simulink model "model5"  (R2022a)
settings: Solver=FixedStepAuto  StartTime=0.0  StopTime=300  FixedStep=1  RelTol=1e-3
values from neighbouring files (symbols this model uses):
  testMap = [0  0  0; 0  1  0; 0  0  0]    [aufgabe2.mat]
settings Model: Creator=JadKHaddad  LastModifiedBy=JadKHaddad

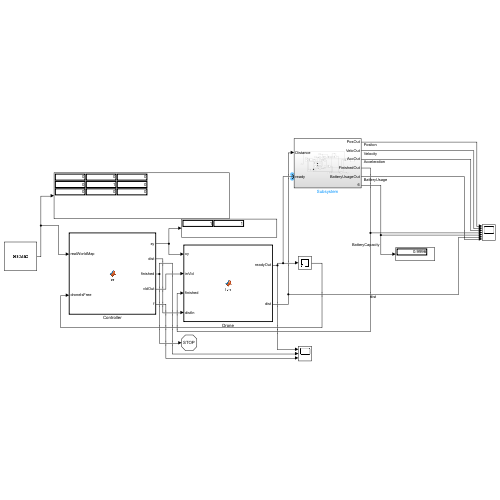
[thumbnail: Simulink's stored preview of the top-level diagram]
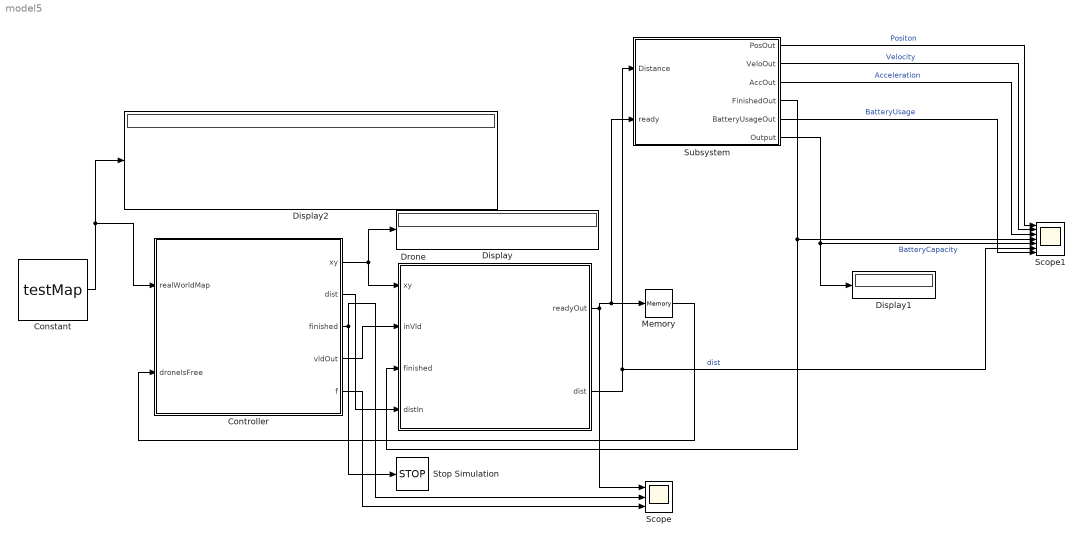
== system model5 ==
  Constant : Constant  Value=testMap  VectorParams1D=off
  Controller : MATLAB Function  TreatAsAtomicUnit=on
  Display : Display
  Display1 : Display
  Display2 : Display
  Drone : MATLAB Function  TreatAsAtomicUnit=on
  Memory : Memory
  Scope : Scope  NumInputPorts=3
  Scope1 : Scope  NumInputPorts=7
  Stop Simulation : Stop
  Subsystem : Subsystem
  wires:
  Drone/1(readyOut) -> Subsystem/2(ready), Memory/1, Scope/1
  Constant/1 -> Display2/1, Controller/1(realWorldMap)
  Controller/1(xy) -> Drone/1(xy), Display/1
  Subsystem/5(BatteryUsageOut) -> Scope1/7  "BatteryUsage"
  Subsystem/4(FinishedOut) -> Drone/3(finished), Scope1/4
  Subsystem/6(Output) -> Display1/1, Scope1/5  "BatteryCapacity"
  Controller/3(finished) -> Scope/2, Stop Simulation/1
  Memory/1 -> Controller/2(droneIsFree)
  Controller/5(f) -> Scope/3
  Subsystem/1(PosOut) -> Scope1/1  "Positon"
  Subsystem/2(VeloOut) -> Scope1/2  "Velocity"
  Controller/4(vldOut) -> Drone/2(inVld)
  Subsystem/3(AccOut) -> Scope1/3  "Acceleration"
  Drone/2(dist) -> Scope1/6, Subsystem/1(Distance)  "dist"
  Controller/2(dist) -> Drone/4(distIn)

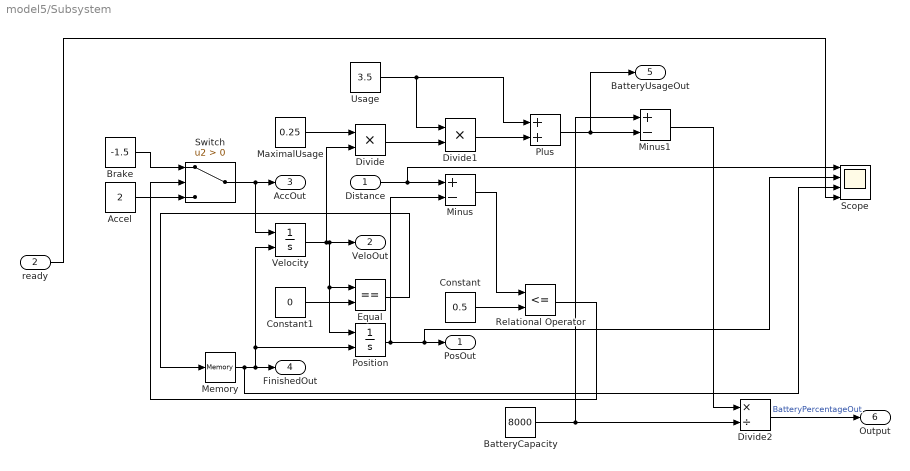
== system model5/Subsystem ==
  Distance : Inport
  ready : Inport  Port=2
  Accel : Constant  Value=2
  BatteryCapacity : Constant  Value=8000
  Brake : Constant  Value=-1.5
  Constant : Constant  Value=0.5
  Constant1 : Constant  Value=0
  Divide : Product  Inputs=**  RndMeth=Round
  Divide1 : Product  Inputs=**
  Divide2 : Product  Inputs=*/
  Equal : RelationalOperator  Operator===  OutDataTypeStr=boolean  RndMeth=Simplest  InputSameDT=off
  MaximalUsage : Constant  Value=0.25
  Memory : Memory
  Minus : Sum  Inputs=+-
  Minus1 : Sum  Inputs=+-
  Plus : Sum
  Position : Integrator  ExternalReset=rising
  Relational Operator : RelationalOperator  Operator=<=  OutDataTypeStr=boolean  RndMeth=Simplest  InputSameDT=off
  Scope : Scope  NumInputPorts=4
  Switch : Switch  Criteria=u2 > Threshold  SaturateOnIntegerOverflow=off  InputSameDT=off
  Usage : Constant  Value=3.5
  Velocity : Integrator  ExternalReset=rising  LimitOutput=on  UpperSaturationLimit=1  LowerSaturationLimit=0
  PosOut : Outport
  VeloOut : Outport  Port=2
  AccOut : Outport  Port=3
  FinishedOut : Outport  Port=4
  BatteryUsageOut : Outport  Port=5
  Output : Outport  Port=6
  wires:
  Position/1 -> Minus/2, Scope/2, PosOut/1
  Relational Operator/1 -> Switch/2
  Minus1/1 -> Divide2/1
  Divide2/1 -> Output/1  "BatteryPercentageOut"
  MaximalUsage/1 -> Divide/1
  Divide/1 -> Divide1/2
  Divide1/1 -> Plus/2
  Memory/1 -> Scope/3, Velocity/2, Position/2, FinishedOut/1
  Distance/1 -> Scope/1, Minus/1
  Constant/1 -> Relational Operator/2
  Constant1/1 -> Equal/2
  Brake/1 -> Switch/1
  Equal/1 -> Memory/1
  Minus/1 -> Relational Operator/1
  Switch/1 -> Velocity/1, AccOut/1
  Accel/1 -> Switch/3
  BatteryCapacity/1 -> Minus1/1, Divide2/2
  Usage/1 -> Plus/1, Divide1/1
  Velocity/1 -> Equal/1, Position/1, VeloOut/1, Divide/2
  Plus/1 -> Minus1/2, BatteryUsageOut/1
  ready/1 -> Scope/4

== matlab function model5/Drone ==
  settings: updateMethod=DISCRETE
  data: xy input; readyOut output; inVld input; finished input; dist output; distIn input
function [readyOut, dist] = fcn(xy, inVld, finished, distIn)

persistent ready
if isempty(ready)
    ready = 1;
end

ready = 0;

if finished == 1
    ready = 1;
end
if inVld == 1 && ready == 1
    ready = 0;
end

dist = distIn;
readyOut = ready;

== matlab function model5/Controller ==
  data: realWorldMap input; xy output; dist output; droneIsFree input; finished output; vldOut output; f output
function [xy, dist, finished, vldOut, f] = fcn(realWorldMap, droneIsFree)
    persistent index
    persistent indexLimit
    persistent path
    persistent lastXY
    


    if isempty(index)
        index = 1;
    end
    if isempty(indexLimit)
        indexLimit = 2;
    end
    if isempty(path)
        path = ones(length(realWorldMap)*length(realWorldMap),2);
    end
    if isempty(lastXY)
        lastXY = [-1 -1];
    end

    
    vldOut = 0;
    finished = 0;
    xy = [1 1];
    dist = -1;
    f = droneIsFree;

    if index >= length(realWorldMap)*length(realWorldMap)
        finished = 1;
        return
    end
    %update path
    x = lastXY(1, 1);
    y = lastXY(1, 2);
    if droneIsFree == 1 && ~isequal(x, -1)
        %update path
        %disp("updating path");

        if realWorldMap(x,y) == 0
            if x + 1 <= length(realWorldMap) && realWorldMap(x + 1, y) == 0 && containsFunc(path, x + 1, y) == 0
                newRow = [x+1 y];
                path(indexLimit,:) = newRow;
                indexLimit = indexLimit + 1;
            end
            
            if y + 1 <= length(realWorldMap) && realWorldMap(x, y + 1) == 0 && containsFunc(path, x, y + 1) == 0
                newRow = [x y+1];
                path(indexLimit,:) = newRow;
                indexLimit = indexLimit + 1;
            end
            
            if x - 1 >= 1 && realWorldMap(x - 1, y) == 0 && containsFunc(path, x - 1, y) == 0
                newRow = [x-1 y];
                path(indexLimit-1,:) = newRow;
                indexLimit = indexLimit + 1;
            end
            
            if y - 1 >= 1 && realWorldMap(x, y-1) == 0 && containsFunc(path, x, y - 1) == 0
                newRow = [x y-1];
                path(indexLimit,:) = newRow;
                indexLimit = indexLimit + 1;
            end
        end
        %disp(path);
        %disp(indexLimit);
    end

    if index < indexLimit
        if droneIsFree == 1
            vldOut = 1;
            %get next pos
            xy = path(index,:);
            sourceRow = lastXY(1);
            if sourceRow == -1
                sourceRow = 1;
            end
            sourceCol = lastXY(2);
            if sourceCol == -1
                sourceCol = 1;
            end
            destRow = xy(1);
            destCol = xy(2);
            dist = minDistanceSimulink(realWorldMap, sourceRow, sourceCol, destRow, destCol);
            disp(dist);
            lastXY = xy;
            index = index + 1;
            
        end
    else
        if droneIsFree == 1
            finished = 1;
        end
    end
